simulink model "modele"  (R2025a)
settings: Solver=VariableStepAuto  StartTime=0.0  StopTime=10.0  RelTol=1e-3
values from neighbouring files (symbols this model uses):
  eta_m = 0.4    [variables_procom.m]
  eta_p = 0.5    [variables_procom.m]
  eta_r = 0.96    [variables_procom.m]
  Je = 0.6    [variables_procom.m]
  Jt = 2.22    [variables_procom.m]
  kd = 0    [variables_procom.m]
  ki = 700    [variables_procom.m]
  kp = 3500    [variables_procom.m]
  m = 0.0    (= 0)    [Hulldyn.m]    (also in variables_procom.m = 250000)
  Pe = 5    [variables_procom.m]
  Re = 1.5    [variables_procom.m]
  Rme = 6.6080    (= 6.608)    [variables_procom.m]
  Rmt = 4.6680    (= 4.668)    [variables_procom.m]
  Rt = 0.0    (= 0)    [Hulldyn.m]    (also in variables_procom.m = 1.8)
  Tc = 0.0    (= 0)    [Hulldyn.m]    (also in variables_procom.m = 1)
undefined symbols (not defined in the file or in its folder): eta_mt, ma, Py
libraries: slpidlib x3
settings Model: Creator=leagr  LastModifiedBy=leagr

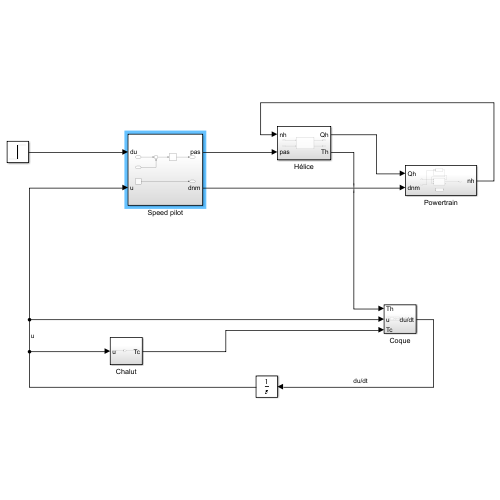
[thumbnail: Simulink's stored preview of the top-level diagram]
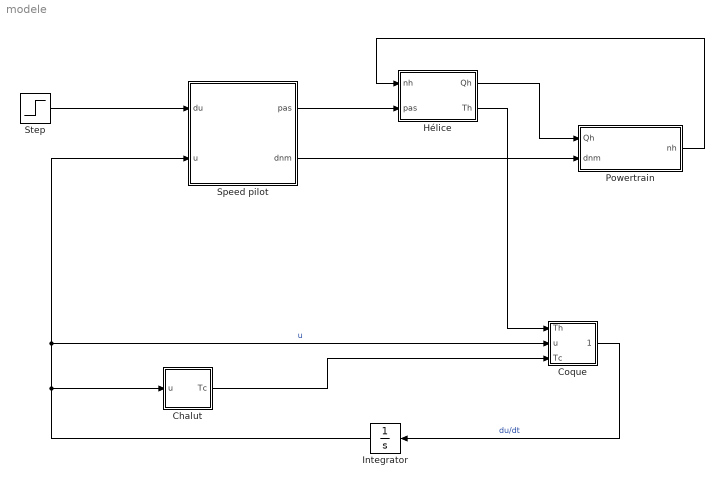
== system modele ==
  Chalut : Subsystem
  Coque : Subsystem
  Hélice : Subsystem
  Integrator : Integrator
  Powertrain : Subsystem
  Speed pilot : Subsystem
  Step : Step  SampleTime=0
  wires:
  Coque/1(du/dt) -> Integrator/1  "du/dt"
  Integrator/1 -> Chalut/1(u), Speed pilot/2(u), Coque/2(u)  "u"
  Chalut/1(Tc) -> Coque/3(Tc)
  Hélice/1(Qh) -> Powertrain/1(Qh)
  Hélice/2(Th) -> Coque/1(Th)
  Powertrain/1(nh) -> Hélice/1(nh)
  Speed pilot/1(pas) -> Hélice/2(pas)
  Speed pilot/2(dnm) -> Powertrain/2(dnm)
  Step/1 -> Speed pilot/1(du)

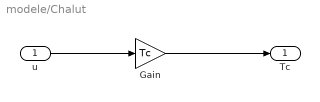
== system modele/Chalut ==
  u : Inport
  Gain : Gain  Gain=Tc
  Tc : Outport
  wires:
  u/1 -> Gain/1
  Gain/1 -> Tc/1

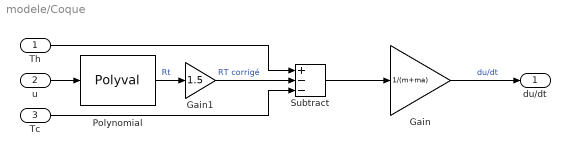
== system modele/Coque ==
  Th : Inport
  u : Inport  Port=2
  Tc : Inport  Port=3
  Gain : Gain  Gain=1/(m+ma)
  Gain1 : Gain  Gain=1.5
  Polynomial : Polyval  Coefs=[768.9,-3894,6949.8,-271.6]
  Subtract : Sum  Inputs=+--
  du/dt : Outport
  wires:
  Th/1 -> Subtract/1
  Subtract/1 -> Gain/1
  Polynomial/1 -> Gain1/1  "Rt"
  Tc/1 -> Subtract/3
  u/1 -> Polynomial/1
  Gain/1 -> du/dt/1  "du/dt"
  Gain1/1 -> Subtract/2  "RT corrigé"

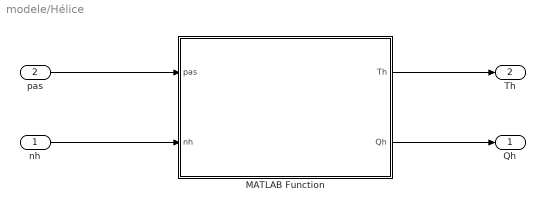
== system modele/Hélice ==
  nh : Inport
  pas : Inport  Port=2
  MATLAB Function : MATLAB Function  TreatAsAtomicUnit=on
  Qh : Outport
  Th : Outport  Port=2
  wires:
  pas/1 -> MATLAB Function/1(pas)
  nh/1 -> MATLAB Function/2(nh)
  MATLAB Function/1(Th) -> Th/1
  MATLAB Function/2(Qh) -> Qh/1

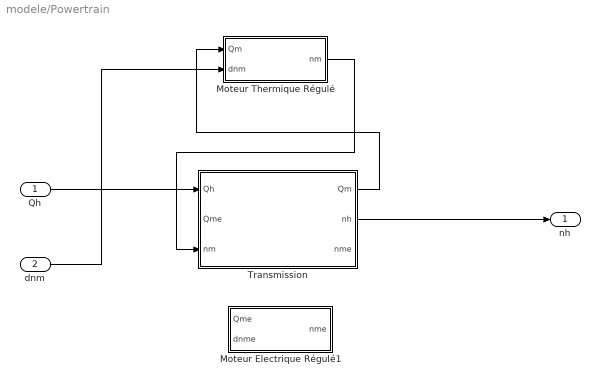
== system modele/Powertrain ==
  Qh : Inport
  dnm : Inport  Port=2
  Moteur Electrique Régulé1 : Subsystem
  Moteur Thermique Régulé : Subsystem
  Transmission : Subsystem
  nh : Outport
  wires:
  Transmission/1(Qm) -> Moteur Thermique Régulé/1(Qm)
  Moteur Thermique Régulé/1(nm) -> Transmission/3(nm)
  Qh/1 -> Transmission/1(Qh)
  Transmission/2(nh) -> nh/1
  dnm/1 -> Moteur Thermique Régulé/2(dnm)

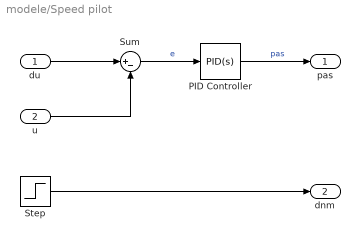
== system modele/Speed pilot ==
  du : Inport
  u : Inport  Port=2
  PID Controller : slpidlib/PID Controller  Controller=PID  Form=Parallel  TimeDomain=Continuous-time  UseExternalTs=off  SampleTime=-1  IntegratorMethod=Forward Euler  FilterMethod=Forward Euler  ControllerParametersSource=internal  P=kp  I=ki  UseKiTs=off  D=kd  UseExternalDerivativeSource=off  N=100  UseFilter=on  TunerSelectOption=Transfer Function Based (PID Tuner App)  InitialConditionSource=internal  InitialConditionForIntegrator=0  InitialConditionForFilter=0  DifferentiatorICPrevScaledInput=0  ExternalReset=none  TrackingMode=off  Kt=1  LimitOutput=off  SatLimitsSource=internal  UpperSaturationLimit=inf  LowerSaturationLimit=-inf  LinearizeAsGain=on  AntiWindupMode=none  Kb=1  LimitIntegrator=off  UpperIntegratorSaturationLimit=inf  LowerIntegratorSaturationLimit=-inf  POutMin=[]  POutMax=[]  IOutMin=[]  IOutMax=[]  DOutMin=[]  DOutMax=[]  NOutMin=[]  NOutMax=[]  SumOutMin=[]  SumOutMax=[]  SaturationOutMin=[]  SaturationOutMax=[]  PParamMin=[]  PParamMax=[]  IParamMin=[]  IParamMax=[]  DParamMin=[]  DParamMax=[]  NParamMin=[]  NParamMax=[]  KbParamMin=[]  KbParamMax=[]  KtParamMin=[]  KtParamMax=[]  KbOutMin=[]  KbOutMax=[]  KtOutMin=[]  KtOutMax=[]  IntegratorOutMin=[]  IntegratorOutMax=[]  FilterOutMin=[]  FilterOutMax=[]  SumI1OutMin=[]  SumI1OutMax=[]  SumI2OutMin=[]  SumI2OutMax=[]  SumI3OutMin=[]  SumI3OutMax=[]  SumI4OutMin=[]  SumI4OutMax=[]  SumDOutMin=[]  SumDOutMax=[]  DifferentiatorOutMin=[]  DifferentiatorOutMax=[]  FilterDiffOutCoefMin=[]  FilterDiffOutCoefMax=[]  ReciprocalOutMin=[]  ReciprocalOutMax=[]  SumDenOutMin=[]  SumDenOutMax=[]  SumNumOutMin=[]  SumNumOutMax=[]  DivideOutMin=[]  DivideOutMax=[]  UdiffTsProdOutMin=[]  UdiffTsProdOutMax=[]  NTsProdOutMin=[]  NTsProdOutMax=[]  UintegralTsProdOutMin=[]  UintegralTsProdOutMax=[]  UngainTsProdOutMin=[]  UngainTsProdOutMax=[]  ClampingZeroOutDataTypeStr=Inherit: Inherit via back propagation  ClampingZeroOutMin=[]  ClampingZeroOutMax=[]  FilterDenConstantOutDataTypeStr=Inherit: Inherit via back propagation  FilterDenConstantOutMin=[]  FilterDenConstantOutMax=[]  PCopyOutDataTypeStr=Inherit: Inherit via back propagation  PCopyOutMin=[]  PCopyOutMax=[]  NCopyOutDataTypeStr=Inherit: Inherit via back propagation  NCopyOutMin=[]  NCopyOutMax=[]  IntegratorContinuousStateAttributes=''  IntegratorStateMustResolveToSignalObject=off  IntegratorRTWStateStorageClass=Auto  FilterContinuousStateAttributes=''  FilterStateMustResolveToSignalObject=off  FilterRTWStateStorageClass=Auto  ParallelPVariant=InternalParameters  IdealPVariant=Disabled  IVariant=InternalParameters  DVariant=InternalParameters  IntegratorVariant=Continuous  SatVariant=Disabled  AWVariant=Passthrough  PCopyVariant=Disabled  TRVariant=Disabled  FdbkBlocksVariant=Forward  IdealPFdbkVariant=Disabled  SatFdbkVariant=Disabled  DerivativeFilterVariant=ContFilter  NVariant=InternalParameters  NCopyVariant=Disabled  FilterICVariant=InternalICsFilter  IntegratorICVariant=InternalICs  ExternalResetVariant=Disabled  TRSumVariant=Passthrough  SumFdbkVariant=Disabled  SumVariant=Sum_PID  TsampFilterVariant=InternalTs  TsampNgainVariant=Passthrough  TsampIntegralVariant=Disabled_SignalSpec  ExternalSaturationOutDataTypeStr=Inherit: Same as second input  DerivativeSourceVariant=ErrorSignal  PreIntVariant=InternalPreInt
  Step : Step  Time=0  After=700  SampleTime=0
  Sum : Sum  Inputs=|+-
  pas : Outport
  dnm : Outport  Port=2
  wires:
  u/1 -> Sum/2
  Sum/1 -> PID Controller/1  "e"
  PID Controller/1 -> pas/1  "pas"
  du/1 -> Sum/1
  Step/1 -> dnm/1

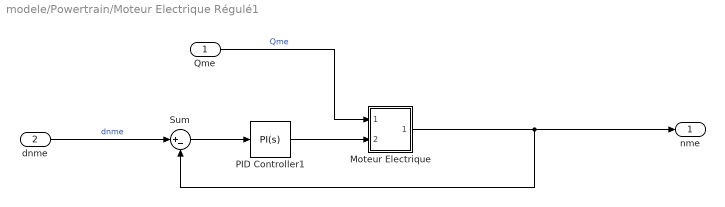
== system modele/Powertrain/Moteur Electrique Régulé1 ==
  Qme : Inport
  dnme : Inport  Port=2
  Moteur Electrique : Subsystem
  PID Controller1 : slpidlib/PID Controller  Controller=PI  Form=Parallel  TimeDomain=Continuous-time  UseExternalTs=off  SampleTime=-1  IntegratorMethod=Forward Euler  FilterMethod=Forward Euler  ControllerParametersSource=internal  P=29.9781477943651  I=96.5900457001455  UseKiTs=off  D=-0.0550740618748937  UseExternalDerivativeSource=off  N=57.1413988020802  UseFilter=on  TunerSelectOption=Transfer Function Based (PID Tuner App)  ZeroCross=off  InitialConditionSource=internal  InitialConditionForIntegrator=0  InitialConditionForFilter=0  DifferentiatorICPrevScaledInput=0  ExternalReset=none  TrackingMode=off  Kt=1  LimitOutput=off  SatLimitsSource=internal  UpperSaturationLimit=inf  LowerSaturationLimit=-inf  LinearizeAsGain=on  AntiWindupMode=none  Kb=1  LimitIntegrator=off  UpperIntegratorSaturationLimit=inf  LowerIntegratorSaturationLimit=-inf  POutMin=[]  POutMax=[]  IOutMin=[]  IOutMax=[]  DOutMin=[]  DOutMax=[]  NOutMin=[]  NOutMax=[]  SumOutMin=[]  SumOutMax=[]  SaturationOutMin=[]  SaturationOutMax=[]  PParamMin=[]  PParamMax=[]  IParamMin=[]  IParamMax=[]  DParamMin=[]  DParamMax=[]  NParamMin=[]  NParamMax=[]  KbParamMin=[]  KbParamMax=[]  KtParamMin=[]  KtParamMax=[]  KbOutMin=[]  KbOutMax=[]  KtOutMin=[]  KtOutMax=[]  IntegratorOutMin=[]  IntegratorOutMax=[]  FilterOutMin=[]  FilterOutMax=[]  SumI1OutMin=[]  SumI1OutMax=[]  SumI2OutMin=[]  SumI2OutMax=[]  SumI3OutMin=[]  SumI3OutMax=[]  SumI4OutMin=[]  SumI4OutMax=[]  SumDOutMin=[]  SumDOutMax=[]  DifferentiatorOutMin=[]  DifferentiatorOutMax=[]  FilterDiffOutCoefMin=[]  FilterDiffOutCoefMax=[]  ReciprocalOutMin=[]  ReciprocalOutMax=[]  SumDenOutMin=[]  SumDenOutMax=[]  SumNumOutMin=[]  SumNumOutMax=[]  DivideOutMin=[]  DivideOutMax=[]  UdiffTsProdOutMin=[]  UdiffTsProdOutMax=[]  NTsProdOutMin=[]  NTsProdOutMax=[]  UintegralTsProdOutMin=[]  UintegralTsProdOutMax=[]  UngainTsProdOutMin=[]  UngainTsProdOutMax=[]  ClampingZeroOutDataTypeStr=Inherit: Inherit via back propagation  ClampingZeroOutMin=[]  ClampingZeroOutMax=[]  FilterDenConstantOutDataTypeStr=Inherit: Inherit via back propagation  FilterDenConstantOutMin=[]  FilterDenConstantOutMax=[]  PCopyOutDataTypeStr=Inherit: Inherit via back propagation  PCopyOutMin=[]  PCopyOutMax=[]  NCopyOutDataTypeStr=Inherit: Inherit via back propagation  NCopyOutMin=[]  NCopyOutMax=[]  IntegratorContinuousStateAttributes=''  IntegratorStateMustResolveToSignalObject=off  IntegratorRTWStateStorageClass=Auto  FilterContinuousStateAttributes=''  FilterStateMustResolveToSignalObject=off  FilterRTWStateStorageClass=Auto  ParallelPVariant=InternalParameters  IdealPVariant=Disabled  IVariant=InternalParameters  DVariant=Disabled  IntegratorVariant=Continuous  SatVariant=Disabled  AWVariant=Passthrough  PCopyVariant=Disabled  TRVariant=Disabled  FdbkBlocksVariant=Forward  IdealPFdbkVariant=Disabled  SatFdbkVariant=Disabled  DerivativeFilterVariant=Disabled  NVariant=Disabled  NCopyVariant=Disabled_SignalSpec  FilterICVariant=Disabled  IntegratorICVariant=InternalICs  ExternalResetVariant=Disabled  TRSumVariant=Passthrough  SumFdbkVariant=Disabled  SumVariant=Sum_PI  TsampFilterVariant=InternalTs  TsampNgainVariant=Passthrough  TsampIntegralVariant=Disabled_SignalSpec  ExternalSaturationOutDataTypeStr=Inherit: Same as second input  DerivativeSourceVariant=Disabled  PreIntVariant=InternalPreInt
  Sum : Sum  Inputs=|+-
  nme : Outport
  wires:
  Qme/1 -> Moteur Electrique/1(Qme)  "Qme"
  Moteur Electrique/1(nme) -> nme/1, Sum/2
  dnme/1 -> Sum/1  "dnme"
  PID Controller1/1 -> Moteur Electrique/2(dnme)
  Sum/1 -> PID Controller1/1

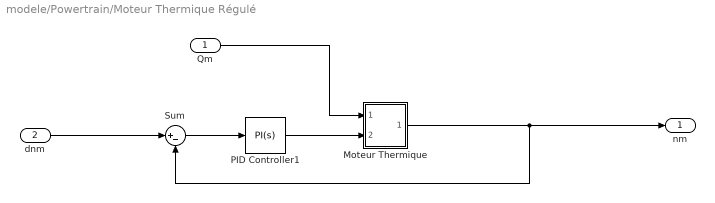
== system modele/Powertrain/Moteur Thermique Régulé ==
  Qm : Inport
  dnm : Inport  Port=2
  Moteur Thermique : Subsystem
  PID Controller1 : slpidlib/PID Controller  Controller=PI  Form=Parallel  TimeDomain=Continuous-time  UseExternalTs=off  SampleTime=-1  IntegratorMethod=Forward Euler  FilterMethod=Forward Euler  ControllerParametersSource=internal  P=7.5474  I=5.2115  UseKiTs=off  D=0  UseExternalDerivativeSource=off  N=100  UseFilter=on  TunerSelectOption=Transfer Function Based (PID Tuner App)  InitialConditionSource=internal  InitialConditionForIntegrator=0  InitialConditionForFilter=0  DifferentiatorICPrevScaledInput=0  ExternalReset=none  TrackingMode=off  Kt=1  LimitOutput=off  SatLimitsSource=internal  UpperSaturationLimit=inf  LowerSaturationLimit=-inf  LinearizeAsGain=on  AntiWindupMode=none  Kb=1  LimitIntegrator=off  UpperIntegratorSaturationLimit=inf  LowerIntegratorSaturationLimit=-inf  POutMin=[]  POutMax=[]  IOutMin=[]  IOutMax=[]  DOutMin=[]  DOutMax=[]  NOutMin=[]  NOutMax=[]  SumOutMin=[]  SumOutMax=[]  SaturationOutMin=[]  SaturationOutMax=[]  PParamMin=[]  PParamMax=[]  IParamMin=[]  IParamMax=[]  DParamMin=[]  DParamMax=[]  NParamMin=[]  NParamMax=[]  KbParamMin=[]  KbParamMax=[]  KtParamMin=[]  KtParamMax=[]  KbOutMin=[]  KbOutMax=[]  KtOutMin=[]  KtOutMax=[]  IntegratorOutMin=[]  IntegratorOutMax=[]  FilterOutMin=[]  FilterOutMax=[]  SumI1OutMin=[]  SumI1OutMax=[]  SumI2OutMin=[]  SumI2OutMax=[]  SumI3OutMin=[]  SumI3OutMax=[]  SumI4OutMin=[]  SumI4OutMax=[]  SumDOutMin=[]  SumDOutMax=[]  DifferentiatorOutMin=[]  DifferentiatorOutMax=[]  FilterDiffOutCoefMin=[]  FilterDiffOutCoefMax=[]  ReciprocalOutMin=[]  ReciprocalOutMax=[]  SumDenOutMin=[]  SumDenOutMax=[]  SumNumOutMin=[]  SumNumOutMax=[]  DivideOutMin=[]  DivideOutMax=[]  UdiffTsProdOutMin=[]  UdiffTsProdOutMax=[]  NTsProdOutMin=[]  NTsProdOutMax=[]  UintegralTsProdOutMin=[]  UintegralTsProdOutMax=[]  UngainTsProdOutMin=[]  UngainTsProdOutMax=[]  ClampingZeroOutDataTypeStr=Inherit: Inherit via back propagation  ClampingZeroOutMin=[]  ClampingZeroOutMax=[]  FilterDenConstantOutDataTypeStr=Inherit: Inherit via back propagation  FilterDenConstantOutMin=[]  FilterDenConstantOutMax=[]  PCopyOutDataTypeStr=Inherit: Inherit via back propagation  PCopyOutMin=[]  PCopyOutMax=[]  NCopyOutDataTypeStr=Inherit: Inherit via back propagation  NCopyOutMin=[]  NCopyOutMax=[]  IntegratorContinuousStateAttributes=''  IntegratorStateMustResolveToSignalObject=off  IntegratorRTWStateStorageClass=Auto  FilterContinuousStateAttributes=''  FilterStateMustResolveToSignalObject=off  FilterRTWStateStorageClass=Auto  ParallelPVariant=InternalParameters  IdealPVariant=Disabled  IVariant=InternalParameters  DVariant=Disabled  IntegratorVariant=Continuous  SatVariant=Disabled  AWVariant=Passthrough  PCopyVariant=Disabled  TRVariant=Disabled  FdbkBlocksVariant=Forward  IdealPFdbkVariant=Disabled  SatFdbkVariant=Disabled  DerivativeFilterVariant=Disabled  NVariant=Disabled  NCopyVariant=Disabled_SignalSpec  FilterICVariant=Disabled  IntegratorICVariant=InternalICs  ExternalResetVariant=Disabled  TRSumVariant=Passthrough  SumFdbkVariant=Disabled  SumVariant=Sum_PI  TsampFilterVariant=InternalTs  TsampNgainVariant=Passthrough  TsampIntegralVariant=Disabled_SignalSpec  ExternalSaturationOutDataTypeStr=Inherit: Same as second input  DerivativeSourceVariant=Disabled  PreIntVariant=InternalPreInt
  Sum : Sum  Inputs=|+-
  nm : Outport
  wires:
  Qm/1 -> Moteur Thermique/1(Qm)
  Moteur Thermique/1(nm) -> Sum/2, nm/1
  dnm/1 -> Sum/1
  PID Controller1/1 -> Moteur Thermique/2(dnm)
  Sum/1 -> PID Controller1/1

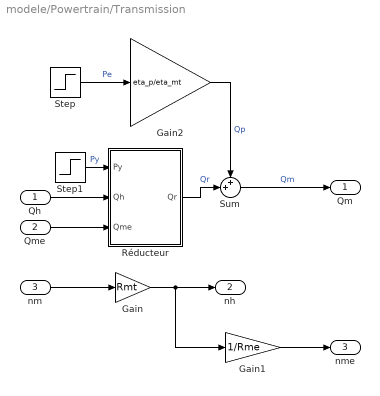
== system modele/Powertrain/Transmission ==
  Qh : Inport
  Qme : Inport  Port=2
  nm : Inport  Port=3
  Gain : Gain  Gain=Rmt
  Gain1 : Gain  Gain=1/Rme
  Gain2 : Gain  Gain=eta_p/eta_mt
  Réducteur : Subsystem
  Step : Step  Time=0  After=Pe  SampleTime=0
  Step1 : Step  Time=0  After=Py  SampleTime=0
  Sum : Sum  Inputs=++|
  Qm : Outport
  nh : Outport  Port=2
  nme : Outport  Port=3
  wires:
  Gain2/1 -> Sum/1  "Qp"
  Step1/1 -> Réducteur/1(Py)  "Py"
  Qh/1 -> Réducteur/2(Qh)
  Step/1 -> Gain2/1  "Pe"
  Sum/1 -> Qm/1  "Qm"
  Réducteur/1(Qr) -> Sum/2  "Qr"
  Qme/1 -> Réducteur/3(Qme)
  Gain1/1 -> nme/1
  Gain/1 -> nh/1, Gain1/1
  nm/1 -> Gain/1

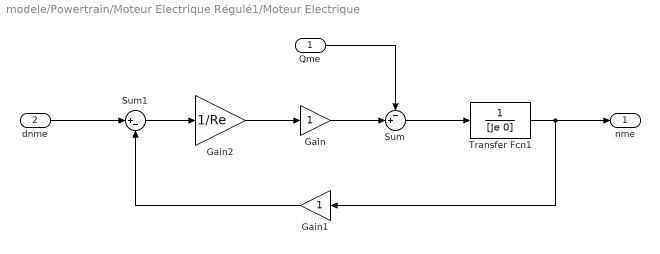
== system modele/Powertrain/Moteur Electrique Régulé1/Moteur Electrique ==
  Qme : Inport
  dnme : Inport  Port=2
  Gain : Gain
  Gain1 : Gain
  Gain2 : Gain  Gain=1/Re
  Sum : Sum  Inputs=-+|
  Sum1 : Sum  Inputs=|+-
  Transfer Fcn1 : TransferFcn  Denominator=[Je 0]
  nme : Outport
  wires:
  Sum/1 -> Transfer Fcn1/1
  Qme/1 -> Sum/1
  Sum1/1 -> Gain2/1
  Gain2/1 -> Gain/1
  Gain/1 -> Sum/2
  dnme/1 -> Sum1/1
  Gain1/1 -> Sum1/2
  Transfer Fcn1/1 -> nme/1, Gain1/1

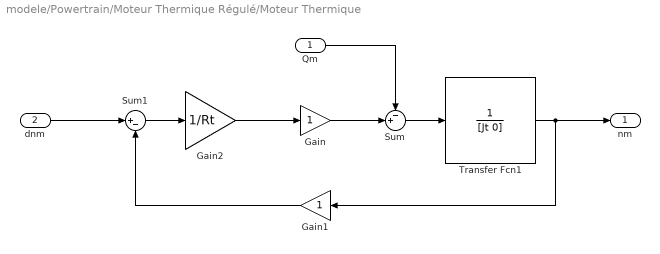
== system modele/Powertrain/Moteur Thermique Régulé/Moteur Thermique ==
  Qm : Inport
  dnm : Inport  Port=2
  Gain : Gain
  Gain1 : Gain
  Gain2 : Gain  Gain=1/Rt
  Sum : Sum  Inputs=-+|
  Sum1 : Sum  Inputs=|+-
  Transfer Fcn1 : TransferFcn  Denominator=[Jt 0]
  nm : Outport
  wires:
  Sum/1 -> Transfer Fcn1/1
  Qm/1 -> Sum/1
  Sum1/1 -> Gain2/1
  Gain2/1 -> Gain/1
  Gain/1 -> Sum/2
  dnm/1 -> Sum1/1
  Gain1/1 -> Sum1/2
  Transfer Fcn1/1 -> Gain1/1, nm/1

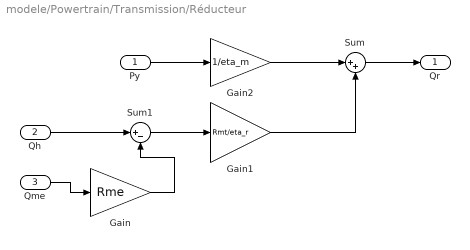
== system modele/Powertrain/Transmission/Réducteur ==
  Py : Inport
  Qh : Inport  Port=2
  Qme : Inport  Port=3
  Gain : Gain  Gain=Rme
  Gain1 : Gain  Gain=Rmt/eta_r
  Gain2 : Gain  Gain=1/eta_m
  Sum : Sum  Inputs=|++
  Sum1 : Sum  Inputs=|+-
  Qr : Outport
  wires:
  Gain2/1 -> Sum/1
  Sum/1 -> Qr/1
  Gain1/1 -> Sum/2
  Py/1 -> Gain2/1
  Qme/1 -> Gain/1
  Gain/1 -> Sum1/2
  Qh/1 -> Sum1/1
  Sum1/1 -> Gain1/1

== matlab function modele/Hélice/MATLAB Function ==
  data: pas input; Th output; nh input; Qh output
function [Th,Qh]= fcn(pas, nh)

;
